simulink model "Thruster_Example_rw"  (R2024b)
settings: Solver=ode4  StartTime=0.0  StopTime=2000  FixedStep=0.01  RelTol=1e-3
undefined symbols (not defined in the file): Cube_L, dt, F_vec, Iws, M_rw, m_tot, norm_Ib, Omega1_init, Omega2_init, Omega3_init, Omega4_init, qb0, rad2rpm, RCS_F, RCS_F_vec, RCS_Pos, RCS_pos, RCS_PWM_Freq, RCS_Sampling_time, RCS_THR_vec, REL_TS_POS_I_0, REL_TS_VEL_I_0, RW_As, RW_Max_Speed, RW_Omegad_max, sat, SC_Ib, SC_state0, SS_Total_Mass, TC_Kepler, THR_dt, THR_Force, THR_freq, THR_Pos, TS_Ib, TS_qb0, TS_state0, TS_wb0, wb0, X, Y, Z
libraries: sm_lib x348, nesl_utility x236, simulink_extras x115, sharedtransform x64, aerolibutil x38, simulink x28, sharedutil x13
(part 3 of 16)

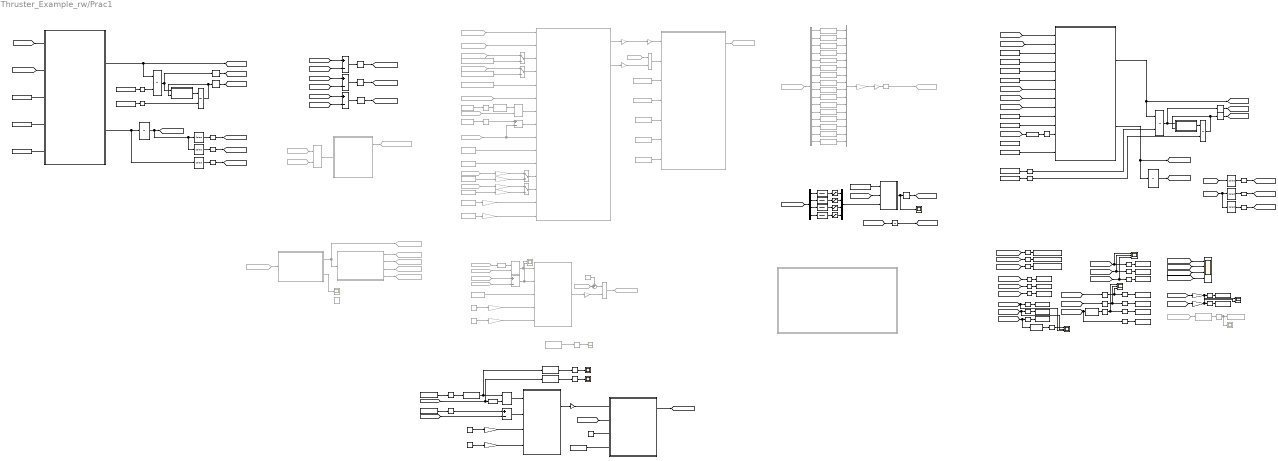
== system Thruster_Example_rw/Prac1 ==
  note: TS 6-DOF Dynamics
  note: RW Model
  note: RW Attitude Controller
  note: Mission Management
  note: SS 6-DOF Dynamics
  note: Relative Vector
  note: RCS Model
  note: Simulation Output
  note: RCS Transition & Attitude Controller
  Add{,1..2,4} (4 alike) : Sum  Inputs=+-
  Add10 : Sum  Commented=on  Inputs=+-
  Add3 : Sum  Commented=on  Inputs=+-
  Constant : Constant  Commented=on  Value=0.3
  Constant1 : Constant  Commented=on  Value=17
  Constant{10,15,27..28,39} (5 alike) : Constant  Value=[0 0 0]'
  Constant11 : Constant  Value=RCS_Pos
  Constant12 : Constant  Value=RCS_THR_vec
  Constant13 : Constant  Value=m_tot
  Constant14 : Constant  Value=RW_Max_Speed
  Constant16 : Constant  Commented=on  Value=100
  Constant17 : Constant  Commented=on  Value=2000
  Constant18 : Constant  Commented=on
  Constant19 : Constant  Value=20
  Constant2 : Constant  Commented=on  Value=200
  Constant20 : Constant  Commented=on  Value=m_tot
  Constant21 : Constant  Value=1000
  Constant22 : Constant  Value=0.01
  Constant23 : Constant  Commented=on  Value=[0 0 0]'
  Constant24 : Constant  Value=RW_Max_Speed
  Constant3 : Constant  Commented=on  Value=2000
  Constant32 : Constant  Commented=on  Value=RW_As
  Constant36 : Constant  Value=TS_Ib
  Constant4 : Constant  Value=SC_Ib
  Constant40 : Constant  Value=TS_wb0
  Constant41 : Constant  Value=TS_qb0
  Constant49 : Constant  Commented=on  Value=[5.0 0 0]'
  Constant5 : Constant  Value=Iws
  Constant52 : Constant  Commented=on  Value=[0 0 0]'
  Constant53 : Constant  Commented=on  Value=SC_Ib
  Constant55 : Constant  Commented=on
  Constant56 : Constant  Commented=on  Value=0.5
  Constant57 : Constant  Commented=on  Value=0.5
  Constant58 : Constant  Commented=on  Value=[0 0 0]
  Constant59 : Constant  Commented=on  Value=[0 0 0]
  Constant6 : Constant  Value=RW_As
  Constant60 : Constant  Commented=on  Value=RCS_Pos
  Constant61 : Constant  Commented=on  Value=RCS_THR_vec
  Constant7 : Constant  Value=[0 0 0.5]'
  Constant8 : Constant  Value=wb0
  Constant9 : Constant  Value=qb0
  Degrees to Radians : simulink_extras/Transformations/Degrees to Radians
  Degrees to Radians1 : simulink_extras/Transformations/Degrees to Radians
  Degrees to Radians2 : simulink_extras/Transformations/Degrees to Radians  Commented=on
  Degrees to Radians3 : simulink_extras/Transformations/Degrees to Radians  Commented=on
  Demux : Demux  Commented=on  Outputs=16
  Demux1 : Demux
  From10 : From  Commented=on  GotoTag=LoS_Quaternion
  From24 : From  Commented=on  GotoTag=mission_flag  TagVisibility=global
  From25 : From  Commented=on  GotoTag=mission_flag  TagVisibility=global
  From30 : From  Commented=on  GotoTag=TS_wb
  From31 : From  Commented=on  GotoTag=TS_q
  From32 : From  Commented=on  GotoTag=q
  From36 : From  Commented=on  GotoTag=q
  From40 : From  Commented=on  GotoTag=wb
  From43 : From  Commented=on  GotoTag=REL_TS_POS_I
  From44 : From  Commented=on  GotoTag=REL_TS_POS_I
  From49 : From  Commented=on  GotoTag=REL_TS_VEL_I
  From53 : From  Commented=on  GotoTag=q
  From55 : From  Commented=on  GotoTag=wb
  From57 : From  Commented=on  GotoTag=REL_TS_POS_I
  From58 : From  Commented=on  GotoTag=RCS_PWPF_CMD
  From59 : From  Commented=on  GotoTag=rel_p_cmd  TagVisibility=global
  From60 : From  Commented=on  GotoTag=LoS_Quaternion
  From63 : From  Commented=on  GotoTag=rel_v_cmd  TagVisibility=global
  From64 : From  Commented=on  GotoTag=Kp_pos  TagVisibility=global
  From65 : From  Commented=on  GotoTag=Kd_pos  TagVisibility=global
  Gain : Gain
  Gain{1,3,5..7,9,18,20} (8 alike) : Gain  Commented=on  Gain=norm_Ib
  Gain{2,10,12,23} (4 alike) : Gain  Commented=on
  Gain11 : Gain  Gain=rad2rpm
  Gain13 : Gain  Gain=norm_Ib
  Gain14 : Gain  Gain=norm_Ib
  Gain22 : Gain  Commented=on  Gain=-1
  Gain4 : Gain  Commented=on  Gain=RCS_F
  Gain8 : Gain  Gain=rad2rpm
  Get LOS Quaternion : MATLAB Function  Commented=on  TreatAsAtomicUnit=on
  Goto : Goto  Commented=on  GotoTag=rel_p_cmd  TagVisibility=global
  Goto12 : Goto  Commented=on  GotoTag=Kd_pos  TagVisibility=global
  Goto23 : Goto  Commented=on  GotoTag=RCS_mea
  Goto26 : Goto  Commented=on  GotoTag=mission_flag  TagVisibility=global
  Goto3 : Goto  Commented=on  GotoTag=RCS_PWPF_CMD
  Goto32 : Goto  Commented=on  GotoTag=RW_torque_cmd
  Goto34 : Goto  Commented=on  GotoTag=LoS_Quaternion
  Goto4 : Goto  Commented=on  GotoTag=rel_v_cmd  TagVisibility=global
  Goto5 : Goto  Commented=on  GotoTag=Kp_pos  TagVisibility=global
  Inetial to body : aerolibutil/Quaternion Rotation  Commented=on
  Integrator : Integrator  InitialConditionSource=external  InitialCondition=wb0
  Integrator2 : Integrator  InitialConditionSource=external  InitialCondition=wb0
  Integrator3 : Integrator  InitialCondition=[Omega1_init Omega2_init Omega3_init Omega4_init]'
  Integrator4 : Integrator  InitialConditionSource=external
  Integrator5 : Integrator  InitialCondition=TS_state0'
  Integrator7 : Integrator  InitialConditionSource=external
  Integrator8 : Integrator  InitialCondition=SC_state0'
  Los angle : Scope  Commented=on
  Manual Switch{,1,3..4} (4 alike) : ManualSwitch  Commented=on
  Mission_Supporter : MATLAB Function  Commented=on  TreatAsAtomicUnit=on
  Mux1 : Mux
  Mux2 : Mux  Commented=on  Inputs=16
  PWM{,1..15} (16 alike) : simulink/Discontinuities/PWM  Commented=on  DisableCoverage=on  Period=RCS_PWM_Freq  InitialDelay=0  DisallowZeroDutyCycle=off  RunAtFixedTimeIntervals=on  SampleTime=RCS_Sampling_time
  Product : Product  Commented=on
  Product1 : Product  Commented=on
  QP Opt : MATLAB Function  TreatAsAtomicUnit=on
  Quaternion Inverse : aerolibutil/Quaternion Inverse  Commented=on
  Quaternion Inverse2 : aerolibutil/Quaternion Inverse
  Quaternion Multiplication1 : aerolibutil/Quaternion Multiplication  Commented=on
  Quaternion Multiplication2 : aerolibutil/Quaternion Multiplication
  Quaternion Multiplication4 : aerolibutil/Quaternion Multiplication  Commented=on
  Quaternion_Kinematics : MATLAB Function  TreatAsAtomicUnit=on
  Quaternion_Kinematics1 : MATLAB Function  TreatAsAtomicUnit=on
  Quaternions to Direction Cosine Matrix : sharedtransform/Quaternions to  Direction Cosine Matrix  aMode=aMode
      settings: LibrarySourceBlock=|
      | aerolibtransform2/Quaternions to
      | Direction Cosine Matrix
  Quaternions to Rotation Angles{,1,4..5} (4 alike) : sharedtransform/Quaternions to Rotation Angles  rotationOrder=ZYX  aMode=aMode
  Quaternions to Rotation Angles2 : sharedtransform/Quaternions to Rotation Angles  Commented=on  rotationOrder=ZYX  aMode=aMode
  Quaternions to Rotation Angles3 : sharedtransform/Quaternions to Rotation Angles  Commented=on  rotationOrder=ZYX  aMode=aMode
  RCS_Position&Attitude_Controller : MATLAB Function  Commented=on  TreatAsAtomicUnit=on
  RCS_Relative_Position_Control_Allocation2 : MATLAB Function  Commented=on  TreatAsAtomicUnit=on
  RW_torque_cmd : Scope
  Radians to Degrees{,1..3,6..7} (6 alike) : simulink_extras/Transformations/Radians to Degrees
  Radians to Degrees4 : simulink_extras/Transformations/Radians to Degrees  Commented=on
  Radians to Degrees5 : simulink_extras/Transformations/Radians to Degrees  Commented=on
  Rel transition / flag : Scope  NumInputPorts=4
  Reshape{,1..2,12..13,19..23} (10 alike) : Reshape  OutputDimensionality=Column vector (2-D)
  Reshape{3..11,15..18,24..28} (18 alike) : Reshape  OutputDimensionality=Row vector (2-D)
  Reshape14 : Reshape  Commented=on  OutputDimensionality=Column vector (2-D)
  Rotation Angles to Quaternions : sharedtransform/Rotation Angles to Quaternions  rotationOrder=ZYX  aMode=aMode
  Rotation Angles to Quaternions2 : sharedtransform/Rotation Angles to Quaternions  Commented=on  rotationOrder=ZYX  aMode=aMode
  SC 6-DOF Dynamics : MATLAB Function  TreatAsAtomicUnit=on
  SS Attitude Control wrt ECI : MATLAB Function  Commented=on  TreatAsAtomicUnit=on
  SS attitude : Scope  NumInputPorts=3
  SS transition : Scope  NumInputPorts=3
  Saturation{1..4} (4 alike) : Saturate  UpperLimit=RW_Omegad_max  LowerLimit=-RW_Omegad_max
  Scope : Scope  Commented=on
  Scope1 : Scope  Commented=on
  Scope2 : Scope
  Scope3 : Scope
  Selector1 : Selector  InputPortWidth=6  IndexOptions=Index vector (dialog)  Indices=[1 2 3]  OutputSizes=1
  Selector2 : Selector  InputPortWidth=6  IndexOptions=Index vector (dialog)  Indices=[4 5 6]  OutputSizes=1
  Selector6 : Selector  InputPortWidth=6  IndexOptions=Index vector (dialog)  Indices=[1 2 3]  OutputSizes=1
  Selector7 : Selector  InputPortWidth=6  IndexOptions=Index vector (dialog)  Indices=[1 2 3]  OutputSizes=1
  Selector8 : Selector  InputPortWidth=6  IndexOptions=Index vector (dialog)  Indices=[4 5 6]  OutputSizes=1
  Selector9 : Selector  InputPortWidth=6  IndexOptions=Index vector (dialog)  Indices=[4 5 6]  OutputSizes=1
  Simple PD Control : MATLAB Function  TreatAsAtomicUnit=on
  Stop Simulation : Stop  Commented=on
  Subsystem : Subsystem  Commented=on
  Sum : Sum  Commented=on  Inputs=-+|
  TS 6-DOF Dynamics : MATLAB Function  TreatAsAtomicUnit=on
  Target attitude : Scope  NumInputPorts=3
  To Workspace : ToWorkspace  VariableName=SS_POS_I  SampleTime=-1
      settings: Save2DSignal=2-D array (concatenate along first dimension)
  To Workspace1 : ToWorkspace  VariableName=SS_VEL_I  SampleTime=-1
      settings: Save2DSignal=2-D array (concatenate along first dimension)
  To Workspace10 : ToWorkspace  VariableName=TS_VEL_I  SampleTime=-1
      settings: Save2DSignal=2-D array (concatenate along first dimension)
  To Workspace11 : ToWorkspace  VariableName=TS_ACC_I  SampleTime=-1
      settings: Save2DSignal=2-D array (concatenate along first dimension)
  To Workspace12 : ToWorkspace  VariableName=SS_q_b  SampleTime=-1
      settings: Save2DSignal=2-D array (concatenate along first dimension)
  To Workspace13 : ToWorkspace  VariableName=TS_wb  SampleTime=-1
      settings: Save2DSignal=2-D array (concatenate along first dimension)
  To Workspace14 : ToWorkspace  VariableName=wheel_rate  SampleTime=-1
      settings: Save2DSignal=2-D array (concatenate along first dimension)
  To Workspace15 : ToWorkspace  VariableName=TS_q  SampleTime=-1
      settings: Save2DSignal=2-D array (concatenate along first dimension)
  To Workspace16 : ToWorkspace  VariableName=TS_wd  SampleTime=-1
      settings: Save2DSignal=2-D array (concatenate along first dimension)
  To Workspace17 : ToWorkspace  Commented=on  VariableName=LoS_angle  SampleTime=-1
      settings: Save2DSignal=2-D array (concatenate along first dimension)
  To Workspace18 : ToWorkspace  VariableName=wheel_rated  SampleTime=-1
      settings: Save2DSignal=2-D array (concatenate along first dimension)
  To Workspace2 : ToWorkspace  VariableName=SS_ACC_I  SampleTime=-1
      settings: Save2DSignal=2-D array (concatenate along first dimension)
  To Workspace3 : ToWorkspace  VariableName=SS_wd_b  SampleTime=-1
      settings: Save2DSignal=2-D array (concatenate along first dimension)
  To Workspace4 : ToWorkspace  VariableName=SS_w_b  SampleTime=-1
      settings: Save2DSignal=2-D array (concatenate along first dimension)
  To Workspace5 : ToWorkspace  VariableName=SS_angle_I  SampleTime=-1
      settings: Save2DSignal=2-D array (concatenate along first dimension)
  To Workspace6 : ToWorkspace  VariableName=REL_TS_POS_I  SampleTime=-1
      settings: Save2DSignal=2-D array (concatenate along first dimension)
  To Workspace7 : ToWorkspace  VariableName=REL_TS_VEL_I  SampleTime=-1
      settings: Save2DSignal=2-D array (concatenate along first dimension)
  To Workspace8 : ToWorkspace  VariableName=REL_TS_ACC_I  SampleTime=-1
      settings: Save2DSignal=2-D array (concatenate along first dimension)
  To Workspace9 : ToWorkspace  VariableName=TS_POS_I  SampleTime=-1
      settings: Save2DSignal=2-D array (concatenate along first dimension)
  Transfer Fcn{,1..3} (4 alike) : TransferFcn  Numerator=[10]  Denominator=[1 10]
  Transport Delay1 : TransportDelay  DelayTime=dt  InitialOutput=qb0
  Transport Delay2 : TransportDelay  DelayTime=dt  InitialOutput=wb0
  Transport Delay3 : TransportDelay  DelayTime=dt  InitialOutput=[0 0 0]'
  Transport Delay4 : TransportDelay  DelayTime=dt  InitialOutput=REL_TS_VEL_I_0
  Transport Delay5 : TransportDelay  DelayTime=dt  InitialOutput=REL_TS_POS_I_0
  Transport Delay6 : TransportDelay  DelayTime=dt  InitialOutput=[0 0 0 0]'
  Transport Delay7 : TransportDelay  DelayTime=dt  InitialOutput=TS_qb0
  Transport Delay8 : TransportDelay  DelayTime=dt  InitialOutput=TS_wb0
  Transpose : Math  Operator=transpose
  attitude error : Scope  Commented=on  NumInputPorts=2
  command_generator : MATLAB Function  Commented=on  TreatAsAtomicUnit=on
  saturation : MATLAB Function  TreatAsAtomicUnit=on
  wheel rate : Scope  NumInputPorts=2
  wires:
  [q] -> Reshape3/1, Quaternions to Rotation Angles/1
  [q] -> Quaternions to Direction Cosine Matrix/1
  Radians to Degrees2/1 -> SS attitude/1, Reshape11/1
  SC 6-DOF Dynamics/1(wd) -> Integrator/1, [wd]
  Add/1 -> Transport Delay5/1
  Add1/1 -> Transport Delay4/1
  [SS_v_I] -> Add1/2
  Reshape7/1 -> To Workspace1/1
  Constant5/1 -> SC 6-DOF Dynamics/5(Iws)
  Mux1/1 -> saturation/3(torque_cmd)
  Reshape28/1 -> To Workspace18/1
  Radians to Degrees1/1 -> SS attitude/2, Reshape10/1
  SC 6-DOF Dynamics/2(xd) -> Integrator8/1, [xd]
  Gain23/1 -> Product/2
  Gain8/1 -> wheel rate/2, Reshape28/1
  [Omegad_mea] -> Integrator3/1
  PWM7/1 -> Mux2/8
  PWM4/1 -> Mux2/5
  PWM6/1 -> Mux2/7
  PWM/1 -> Mux2/1
  Demux/4 -> PWM3/1
  Mux2/1 -> Gain4/1
  Demux/3 -> PWM2/1
  [SS_a_I] -> Add2/2
  Selector6/1 -> Reshape/1
  Gain10/1 -> Product1/2
  [TS_a_I] -> Reshape26/1
  Reshape4/1 -> To Workspace16/1
  From32/1 -> Quaternion Multiplication1/2
  From55/1 -> Add3/2, RCS_Position&Attitude_Controller/9(wb)
  Transport Delay8/1 -> [TS_wb]
  Add3/1 -> RCS_Position&Attitude_Controller/8("w_err ")
  Radians to Degrees3/1 -> Target attitude/1
  [TS_p_I] -> Reshape24/1
  Product1/1 -> Goto32/1
  Constant61/1 -> RCS_Relative_Position_Control_Allocation2/4(RCS_F_vec)
  From64/1 -> Gain1/1
  Constant18/1 -> Sum/1
  From59/1 -> Manual Switch/1
  Selector7/1 -> Reshape1/1
  Quaternions to Rotation Angles1/1 -> Radians to Degrees3/1
  Demux/1 -> PWM/1
  Constant40/1 -> Reshape12/1
  Quaternion Inverse/1 -> Quaternion Multiplication1/1
  Reshape9/1 -> To Workspace3/1
  [SS_p_I] -> Add/2
  Constant16/1 -> Gain6/1
  From58/1 -> Demux/1
  Radians to Degrees4/1 -> To Workspace17/1, Los angle/1
  From25/1 -> Sum/2
  Demux/9 -> PWM8/1
  Constant1/1 -> Gain18/1
  Gain6/1 -> SS Attitude Control wrt ECI/4(Kp_rw)
  Degrees to Radians2/1 -> Rotation Angles to Quaternions2/1
  Gain20/1 -> Manual Switch3/2
  From30/1 -> Add10/2
  Constant39/1 -> TS 6-DOF Dynamics/4(T_ext)
  Reshape16/1 -> To Workspace6/1
  Gain5/1 -> Manual Switch4/1
  Manual Switch3/1 -> RCS_Position&Attitude_Controller/12(Kp_pos)
  [TS_q] -> Quaternions to Rotation Angles1/1, Reshape15/1
  Reshape8/1 -> To Workspace2/1
  From57/1 -> Mission_Supporter/1(res_pos)
  Gain9/1 -> SS Attitude Control wrt ECI/5(Kd_rw)
  [TS_v_I] -> Add1/1
  Demux/16 -> PWM15/1
  [Omegad_mea] -> SC 6-DOF Dynamics/8(Omegad)
  Reshape5/1 -> To Workspace13/1
  Constant6/1 -> SC 6-DOF Dynamics/6(As)
  Demux/5 -> PWM4/1
  command_generator/1(rel_p_cmd) -> Goto/1
  Demux/11 -> PWM10/1
  Selector8/1 -> Reshape2/1
  Demux1/3 -> Transfer Fcn2/1
  Manual Switch/1 -> RCS_Position&Attitude_Controller/3(r_ref)
  Gain1/1 -> Manual Switch3/1
  From10/1 -> Quaternions to Rotation Angles3/1
  Constant8/1 -> Reshape19/1
  Constant10/1 -> SC 6-DOF Dynamics/14(F_ext)
  Manual Switch1/1 -> RCS_Position&Attitude_Controller/4(v_ref)
  Reshape25/1 -> To Workspace10/1
  Gain18/1 -> Manual Switch4/2
  Gain2/1 -> Gain22/1
  command_generator/3(Kp_pos) -> Goto5/1
  [mission_flag] -> Rel transition / flag/4
  Quaternions to Rotation Angles3/1 -> Radians to Degrees4/1
  Constant60/1 -> RCS_Relative_Position_Control_Allocation2/3(RCS_pos)
  Demux/12 -> PWM11/1
  Manual Switch4/1 -> RCS_Position&Attitude_Controller/13(Kd_pos)
  Saturation3/1 -> Mux1/4
  Reshape27/1 -> To Workspace14/1
  Constant57/1 -> RCS_Relative_Position_Control_Allocation2/7(wT)
  command_generator/4(Kd_pos) -> Goto12/1
  [REL_TS_VEL_I] -> Rel transition / flag/2
  Constant23/1 -> RCS_Position&Attitude_Controller/5(a_ref)
  [x] -> Selector6/1
  Constant49/1 -> Manual Switch/2
  From60/1 -> Quaternion Multiplication4/2
  Reshape3/1 -> To Workspace12/1
  Constant52/1 -> Manual Switch1/2
  Demux/13 -> PWM12/1
  Constant53/1 -> RCS_Position&Attitude_Controller/11(Ib)
  Reshape12/1 -> Integrator2/2
  [xd] -> Selector8/1, Selector7/1
  [x] -> SC 6-DOF Dynamics/2(x)
  Radians to Degrees/1 -> SS attitude/3, Reshape9/1
  Constant3/1 -> Gain3/1
  command_generator/2(rel_v_cmd) -> Goto4/1
  Integrator5/1 -> Selector2/1, Selector1/1, [TS_x]
  Reshape14/1 -> Goto23/1
  [REL_TS_POS_I] -> Rel transition / flag/1
  Constant20/1 -> RCS_Position&Attitude_Controller/10(m_sc)
  Transport Delay6/1 -> [Omegad_mea]
  RCS_Position&Attitude_Controller/1(F_cmd_B) -> Gain2/1
  Reshape11/1 -> To Workspace5/1
  Constant55/1 -> RCS_Relative_Position_Control_Allocation2/5(Tmax)
  Gain3/1 -> RCS_Position&Attitude_Controller/15(Kd_att)
  [TS_a_I] -> Add2/1
  Demux/2 -> PWM1/1
  Rotation Angles to Quaternions2/1 -> Quaternion Multiplication4/1
  [TS_wd] -> Target attitude/3, Reshape4/1
  Reshape6/1 -> To Workspace/1
  Constant32/1 -> SS Attitude Control wrt ECI/3(As)
  Demux1/2 -> Transfer Fcn1/1
  [TS_p_I] -> Add/1
  From49/1 -> RCS_Position&Attitude_Controller/2(v_rel)
  Gain11/1 -> wheel rate/1, Reshape27/1
  Degrees to Radians3/1 -> Add3/1
  [Omega_mea] -> Gain11/1
  From65/1 -> Gain5/1
  From31/1 -> Quaternion Inverse/1
  From44/1 -> RCS_Position&Attitude_Controller/1(r_rel)
  RCS_Position&Attitude_Controller/2(tau_cmd_B) -> Gain23/1
  Reshape22/1 -> [TS_v_I]
  PWM2/1 -> Mux2/3
  Selector2/1 -> Reshape22/1
  Gain7/1 -> RCS_Position&Attitude_Controller/14(Kp_att)
  Reshape26/1 -> To Workspace11/1
  [SS_p_I] -> SS transition/1, Reshape6/1
  Demux/14 -> PWM13/1
  Selector9/1 -> Reshape23/1
  Constant9/1 -> Reshape20/1
  Reshape24/1 -> To Workspace9/1
  Reshape19/1 -> Integrator/2
  Reshape15/1 -> To Workspace15/1
  Saturation1/1 -> Mux1/2
  Transport Delay1/1 -> [q]
  Integrator8/1 -> [x]
  [TS_wb] -> TS 6-DOF Dynamics/1(w)
  Reshape23/1 -> [TS_a_I]
  Transport Delay2/1 -> [wb]
  PWM3/1 -> Mux2/4
  Constant12/1 -> SC 6-DOF Dynamics/11(RCS_vec)
  SS Attitude Control wrt ECI/1(RW_cmd) -> Gain10/1
  Transport Delay4/1 -> [REL_TS_VEL_I]
  PWM1/1 -> Mux2/2
  TS 6-DOF Dynamics/1(wd) -> [TS_wd], Integrator2/1
  Demux/7 -> PWM6/1
  Demux1/1 -> Transfer Fcn/1
  Reshape13/1 -> Integrator4/2
  Gain22/1 -> RCS_Relative_Position_Control_Allocation2/1(F_cmd)
  Constant13/1 -> SC 6-DOF Dynamics/4(m_tot)
  Constant36/1 -> TS 6-DOF Dynamics/3(Ib)
  Demux/8 -> PWM7/1
  Demux/15 -> PWM14/1
  [Omega_mea] -> SC 6-DOF Dynamics/7(Omega)
  Selector1/1 -> Reshape21/1
  [TS_wb] -> Target attitude/2, Reshape5/1
  Quaternion_Kinematics1/1(qd) -> Integrator4/1
  Constant/1 -> Gain20/1
  TS 6-DOF Dynamics/2(xd) -> Selector9/1, Integrator5/1
  Integrator4/1 -> Transport Delay7/1, Quaternion_Kinematics1/2(q)
  PWM14/1 -> Mux2/15
  Saturation2/1 -> Mux1/3
  Constant4/1 -> SC 6-DOF Dynamics/3(Ib)
  [TS_x] -> TS 6-DOF Dynamics/2(x)
  Mission_Supporter/1(flag) -> command_generator/1(flag), Goto26/1
  Constant41/1 -> Reshape13/1
  Quaternions to Rotation Angles/1 -> Radians to Degrees2/1
  Constant58/1 -> Degrees to Radians2/1
  PWM5/1 -> Mux2/6
  Saturation4/1 -> Mux1/1
  [TS_v_I] -> Reshape25/1
  Integrator7/1 -> Transport Delay1/1, Quaternion_Kinematics/2(q)
  [SS_a_I] -> SS transition/3, Reshape8/1
  Constant14/1 -> saturation/1(max_speed)
  [Omega_mea] -> saturation/2(Omega_mea)
  Transport Delay7/1 -> [TS_q]
  PWM12/1 -> Mux2/13
  [wb] -> Radians to Degrees1/1
  Transport Delay3/1 -> [REL_TS_ACC_I]
  PWM9/1 -> Mux2/10
  [Omegad_mea] -> Gain8/1
  Demux1/4 -> Transfer Fcn3/1
  From53/1 -> RCS_Position&Attitude_Controller/6("q ")
  Reshape2/1 -> [SS_a_I]
  Gain12/1 -> Reshape14/1
  Transfer Fcn1/1 -> Saturation1/1
  Transfer Fcn2/1 -> Saturation2/1
  Inetial to body/1 -> Get LOS Quaternion/1(r_rel)
  Transfer Fcn3/1 -> Saturation3/1
  Gain4/1 -> Gain12/1
  [REL_TS_ACC_I] -> Reshape18/1
  Integrator2/1 -> Quaternion_Kinematics1/1(w), Transport Delay8/1
  Reshape18/1 -> To Workspace8/1
  From43/1 -> Inetial to body/2
  From63/1 -> Manual Switch1/1
  Transfer Fcn/1 -> Saturation4/1
  Product/1 -> RCS_Relative_Position_Control_Allocation2/2(tau_cmd)
  Add10/1 -> SS Attitude Control wrt ECI/2(w_err), attitude error/2
  [wb] -> SC 6-DOF Dynamics/1(w)
  Constant11/1 -> SC 6-DOF Dynamics/10(RCS_pos)
  Quaternion Multiplication4/1 -> RCS_Position&Attitude_Controller/7(q_err)
  Quaternion Multiplication1/1 -> attitude error/1, SS Attitude Control wrt ECI/1(q_err)
  Constant59/1 -> Degrees to Radians3/1
  Quaternion_Kinematics/1(qd) -> Integrator7/1
  [REL_TS_ACC_I] -> Rel transition / flag/3
  Demux/6 -> PWM5/1
  [REL_TS_VEL_I] -> Reshape17/1
  [SS_v_I] -> SS transition/2, Reshape7/1
  PWM15/1 -> Mux2/16
  Constant17/1 -> Gain9/1
  [REL_TS_POS_I] -> Reshape16/1
  Transpose/1 -> SC 6-DOF Dynamics/12(R_Ib)
  PWM13/1 -> Mux2/14
  Transport Delay5/1 -> [REL_TS_POS_I]
  Constant2/1 -> Gain7/1
  Reshape1/1 -> [SS_v_I]
  Constant56/1 -> RCS_Relative_Position_Control_Allocation2/6(wF)
  saturation/1(res) -> RW_torque_cmd/1, Transport Delay6/1
  Reshape17/1 -> To Workspace7/1
  Add2/1 -> Transport Delay3/1
  Reshape21/1 -> [TS_p_I]
  Reshape20/1 -> Integrator7/2
  PWM11/1 -> Mux2/12
  [wd] -> Radians to Degrees/1
  Demux/10 -> PWM9/1
  Reshape/1 -> [SS_p_I]
  Constant15/1 -> TS 6-DOF Dynamics/5(F_ext)
  Integrator3/1 -> [Omega_mea]
  Sum/1 -> Product1/1
  Mission_Supporter/2(stop) -> Scope/1
  Integrator/1 -> Transport Delay2/1, Quaternion_Kinematics/1(w)
  PWM8/1 -> Mux2/9
  RCS_Relative_Position_Control_Allocation2/1(duty) -> Goto3/1
  [RCS_mea] -> SC 6-DOF Dynamics/9(RCS_mea)
  [RW_torque_cmd] -> Demux1/1
  Reshape10/1 -> To Workspace4/1
  PWM10/1 -> Mux2/11
  Quaternions to Direction Cosine Matrix/1 -> Transpose/1
  From40/1 -> Add10/1
  From24/1 -> Product/1
  From36/1 -> Inetial to body/1
  Get LOS Quaternion/1(q) -> Goto34/1  "LOS quaternion"
  Add4/1 -> Simple PD Control/2(w_err)
  Quaternion Multiplication2/1 -> Simple PD Control/1(q_err)
  [wb] -> Add4/2
  Rotation Angles to Quaternions/1 -> Quaternion Multiplication2/1, Quaternions to Rotation Angles4/1
  [q] -> Quaternions to Rotation Angles5/1, Quaternion Inverse2/1
  Constant21/1 -> Gain14/1
  Constant19/1 -> Gain13/1
  Gain13/1 -> Simple PD Control/3(Kp_rw)
  Gain14/1 -> Simple PD Control/4(Kd_rw)
  Simple PD Control/1(u) -> Gain/1
  Constant22/1 -> QP Opt/3(dt)
  Constant27/1 -> Degrees to Radians/1
  Degrees to Radians/1 -> Rotation Angles to Quaternions/1
  Constant28/1 -> Degrees to Radians1/1
  Degrees to Radians1/1 -> Add4/1
  Quaternions to Rotation Angles2/1 -> Radians to Degrees5/1
  Radians to Degrees5/1 -> Scope1/1
  Gain/1 -> QP Opt/1(tau_des)
  Quaternion Inverse2/1 -> Quaternion Multiplication2/2
  QP Opt/1(u_rw_cmd) -> [RW_torque_cmd]
  [Omega_mea] -> QP Opt/2(Omega_rw)
  Constant24/1 -> QP Opt/4(RW_max_speed)
  Quaternions to Rotation Angles4/1 -> Radians to Degrees6/1
  Radians to Degrees6/1 -> Scope2/1
  Radians to Degrees7/1 -> Scope3/1
  Quaternions to Rotation Angles5/1 -> Radians to Degrees7/1
